simulink model "KF"  (R2021a)
settings: Solver=ode45  StartTime=0.0  StopTime=tt(end)  MaxStep=0.1  RelTol=1e-3  EnableMultiTasking=on
model workspace (MATLAB code in the model file + MAT data in the model file):
  L = 2.5
  v0 = 0
  xe0 = 0
  xn0 = 0
  theta0 = 0
  Ts = 1
  rr = [0 0 0 0 0 0 0 0 0 0 0 0 ... (9404 elements, 9404x1)]
  tt = [0 0.05 0.1 0.15 0.2 0.25 0.3 0.35 0.4 0.45 0.5 0.55 ... (9404 elements, 9404x1)]
  vv = [25 25 25 25 25 25 25 25 25 25 25 25 ... (9404 elements, 9404x1)]
undefined symbols (not defined in the file or in its folder): Discrete, Time
libraries: simulink x4, pid_lib x2, ctrlSharedLib x1
(part 2 of 2)

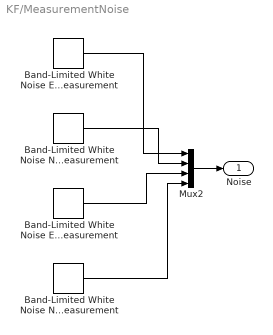
== system KF/MeasurementNoise ==
  Band-Limited White Noise North Position Measurement : simulink/Sources/Band-Limited White Noise  Cov=50  Ts=Ts  seed=[23342]
  Band-Limited White Noise North Velocity Measurement : simulink/Sources/Band-Limited White Noise  Cov=50  Ts=Ts  seed=[23342]
  Band-Limited White Noise East Position Measurement : simulink/Sources/Band-Limited White Noise  Cov=50  Ts=Ts  seed=[23341]
  Band-Limited White Noise East Velocity Measurement : simulink/Sources/Band-Limited White Noise  Cov=50  Ts=Ts  seed=[23341]
  Mux2 : Mux
  Noise : Outport
  wires:
  Mux2/1 -> Noise/1
  Band-Limited White Noise East Position Measurement/1 -> Mux2/1
  Band-Limited White Noise North Position Measurement/1 -> Mux2/2
  Band-Limited White Noise East Velocity Measurement/1 -> Mux2/3
  Band-Limited White Noise North Velocity Measurement/1 -> Mux2/4

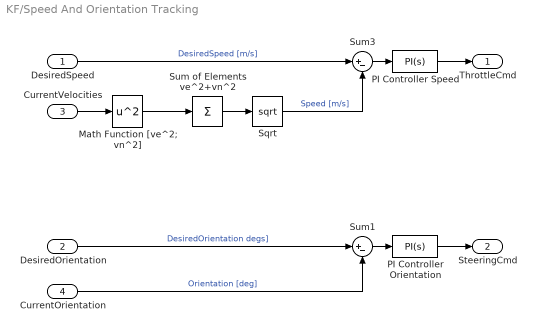
== system KF/Speed And Orientation Tracking ==
  DesiredSpeed : Inport
  DesiredOrientation : Inport  Port=2
  CurrentVelocities : Inport  Port=3
  CurrentOrientation : Inport  Port=4
  Math Function [ve^2; vn^2] : Math  Operator=square  SignedPower=on  SaturateOnIntegerOverflow=on
  PI Controller Orientation : pid_lib/PID Controller  Controller=PI  Form=Parallel  TimeDomain=Continuous-time  UseExternalTs=off  SampleTime=-1  IntegratorMethod=Forward Euler  FilterMethod=Forward Euler  ControllerParametersSource=internal  P=1  I=0.3  D=0  UseFilter=on  N=100  TunerSelectOption=Transfer Function Based (PID Tuner App)  InitialConditionSource=internal  InitialConditionForIntegrator=0  InitialConditionForFilter=0  DifferentiatorICPrevScaledInput=0  ExternalReset=none  TrackingMode=off  Kt=1  LimitOutput=on  SatLimitsSource=internal  UpperSaturationLimit=20  LowerSaturationLimit=-20  LinearizeAsGain=off  AntiWindupMode=clamping  Kb=1  POutMin=[]  POutMax=[]  IOutMin=[]  IOutMax=[]  DOutMin=[]  DOutMax=[]  NOutMin=[]  NOutMax=[]  SumOutMin=[]  SumOutMax=[]  SaturationOutMin=[]  SaturationOutMax=[]  PParamMin=[]  PParamMax=[]  IParamMin=[]  IParamMax=[]  DParamMin=[]  DParamMax=[]  NParamMin=[]  NParamMax=[]  KbParamMin=[]  KbParamMax=[]  KtParamMin=[]  KtParamMax=[]  KbOutMin=[]  KbOutMax=[]  KtOutMin=[]  KtOutMax=[]  IntegratorOutMin=[]  IntegratorOutMax=[]  FilterOutMin=[]  FilterOutMax=[]  SumI1OutMin=[]  SumI1OutMax=[]  SumI2OutMin=[]  SumI2OutMax=[]  SumI3OutMin=[]  SumI3OutMax=[]  SumI4OutMin=[]  SumI4OutMax=[]  SumDOutMin=[]  SumDOutMax=[]  DifferentiatorOutMin=[]  DifferentiatorOutMax=[]  FilterDiffOutCoefMin=[]  FilterDiffOutCoefMax=[]  ReciprocalOutMin=[]  ReciprocalOutMax=[]  SumDenOutMin=[]  SumDenOutMax=[]  SumNumOutMin=[]  SumNumOutMax=[]  DivideOutMin=[]  DivideOutMax=[]  UdiffTsProdOutMin=[]  UdiffTsProdOutMax=[]  NTsProdOutMin=[]  NTsProdOutMax=[]  UintegralTsProdOutMin=[]  UintegralTsProdOutMax=[]  UngainTsProdOutMin=[]  UngainTsProdOutMax=[]  IntegratorContinuousStateAttributes=''  IntegratorStateMustResolveToSignalObject=off  IntegratorRTWStateStorageClass=Auto  FilterContinuousStateAttributes=''  FilterStateMustResolveToSignalObject=off  FilterRTWStateStorageClass=Auto  ParallelPVariant=InternalParameters  IdealPVariant=Disabled  IVariant=InternalParameters  DVariant=Disabled  IntegratorVariant=Continuous  SatVariant=Enabled  AWVariant=ContClampingParallel  PCopyVariant=Disabled  TRVariant=Disabled  FdbkBlocksVariant=Forward  IdealPFdbkVariant=Disabled  SatFdbkVariant=Disabled  DerivativeFilterVariant=Disabled  NVariant=Disabled  NCopyVariant=Disabled_SignalSpec  FilterICVariant=Disabled  IntegratorICVariant=InternalICs  ExternalResetVariant=Disabled  TRSumVariant=Passthrough  SumFdbkVariant=Disabled  SumVariant=Sum_PI  TsampFilterVariant=InternalTs  TsampNgainVariant=Passthrough  TsampIntegralVariant=Passthrough  ExternalSaturationOutDataTypeStr=Inherit: Same as second input
  PI Controller Speed : pid_lib/PID Controller  Controller=PI  Form=Parallel  TimeDomain=Continuous-time  UseExternalTs=off  SampleTime=-1  IntegratorMethod=Forward Euler  FilterMethod=Forward Euler  ControllerParametersSource=internal  P=0.15  I=0.01  D=0  UseFilter=on  N=100  TunerSelectOption=Transfer Function Based (PID Tuner App)  InitialConditionSource=internal  InitialConditionForIntegrator=0  InitialConditionForFilter=0  DifferentiatorICPrevScaledInput=0  ExternalReset=none  TrackingMode=off  Kt=1  LimitOutput=on  SatLimitsSource=internal  UpperSaturationLimit=1  LowerSaturationLimit=-1  LinearizeAsGain=off  AntiWindupMode=clamping  Kb=1  POutMin=[]  POutMax=[]  IOutMin=[]  IOutMax=[]  DOutMin=[]  DOutMax=[]  NOutMin=[]  NOutMax=[]  SumOutMin=[]  SumOutMax=[]  SaturationOutMin=[]  SaturationOutMax=[]  PParamMin=[]  PParamMax=[]  IParamMin=[]  IParamMax=[]  DParamMin=[]  DParamMax=[]  NParamMin=[]  NParamMax=[]  KbParamMin=[]  KbParamMax=[]  KtParamMin=[]  KtParamMax=[]  KbOutMin=[]  KbOutMax=[]  KtOutMin=[]  KtOutMax=[]  IntegratorOutMin=[]  IntegratorOutMax=[]  FilterOutMin=[]  FilterOutMax=[]  SumI1OutMin=[]  SumI1OutMax=[]  SumI2OutMin=[]  SumI2OutMax=[]  SumI3OutMin=[]  SumI3OutMax=[]  SumI4OutMin=[]  SumI4OutMax=[]  SumDOutMin=[]  SumDOutMax=[]  DifferentiatorOutMin=[]  DifferentiatorOutMax=[]  FilterDiffOutCoefMin=[]  FilterDiffOutCoefMax=[]  ReciprocalOutMin=[]  ReciprocalOutMax=[]  SumDenOutMin=[]  SumDenOutMax=[]  SumNumOutMin=[]  SumNumOutMax=[]  DivideOutMin=[]  DivideOutMax=[]  UdiffTsProdOutMin=[]  UdiffTsProdOutMax=[]  NTsProdOutMin=[]  NTsProdOutMax=[]  UintegralTsProdOutMin=[]  UintegralTsProdOutMax=[]  UngainTsProdOutMin=[]  UngainTsProdOutMax=[]  IntegratorContinuousStateAttributes=''  IntegratorStateMustResolveToSignalObject=off  IntegratorRTWStateStorageClass=Auto  FilterContinuousStateAttributes=''  FilterStateMustResolveToSignalObject=off  FilterRTWStateStorageClass=Auto  ParallelPVariant=InternalParameters  IdealPVariant=Disabled  IVariant=InternalParameters  DVariant=Disabled  IntegratorVariant=Continuous  SatVariant=Enabled  AWVariant=ContClampingParallel  PCopyVariant=Disabled  TRVariant=Disabled  FdbkBlocksVariant=Forward  IdealPFdbkVariant=Disabled  SatFdbkVariant=Disabled  DerivativeFilterVariant=Disabled  NVariant=Disabled  NCopyVariant=Disabled_SignalSpec  FilterICVariant=Disabled  IntegratorICVariant=InternalICs  ExternalResetVariant=Disabled  TRSumVariant=Passthrough  SumFdbkVariant=Disabled  SumVariant=Sum_PI  TsampFilterVariant=InternalTs  TsampNgainVariant=Passthrough  TsampIntegralVariant=Passthrough  ExternalSaturationOutDataTypeStr=Inherit: Same as second input
  Sqrt : Sqrt  SaturateOnIntegerOverflow=on
  Sum of Elements ve^2+vn^2 : Sum  Inputs=+
  Sum1 : Sum  Inputs=|+-
  Sum3 : Sum  Inputs=|+-
  ThrottleCmd : Outport
  SteeringCmd : Outport  Port=2
  wires:
  PI Controller Speed/1 -> ThrottleCmd/1
  DesiredSpeed/1 -> Sum3/1  "DesiredSpeed [m/s]"
  Sum3/1 -> PI Controller Speed/1
  CurrentVelocities/1 -> Math Function [ve^2; vn^2]/1
  Math Function [ve^2; vn^2]/1 -> Sum of Elements ve^2+vn^2/1
  Sum of Elements ve^2+vn^2/1 -> Sqrt/1
  Sqrt/1 -> Sum3/2  "Speed [m/s]"
  PI Controller Orientation/1 -> SteeringCmd/1
  DesiredOrientation/1 -> Sum1/1  "DesiredOrientation degs]"
  Sum1/1 -> PI Controller Orientation/1
  CurrentOrientation/1 -> Sum1/2  "Orientation [deg]"

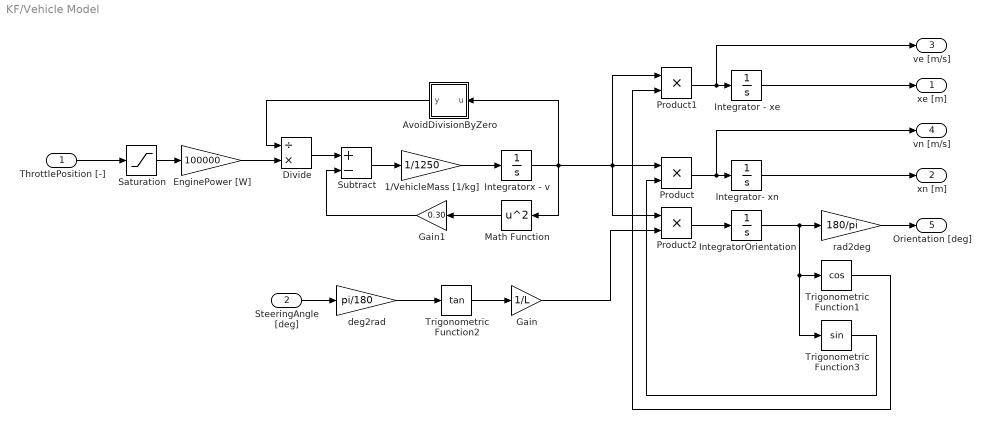
== system KF/Vehicle Model ==
  ThrottlePosition [-] : Inport
  "SteeringAngle [deg] " : Inport  Port=2
  1/VehicleMass [1/kg] : Gain  Gain=1/1250
  AvoidDivisionByZero : Subsystem
  Divide : Product  Inputs=/*
  EnginePower [W] : Gain  Gain=100000
  Gain : Gain  Gain=1/L
  Gain1 : Gain  Gain=0.30
  Integrator - xe : Integrator  InitialCondition=xe0
  Integrator- xn : Integrator  InitialCondition=xn0
  IntegratorOrientation : Integrator  InitialCondition=theta0
  Integratorx - v : Integrator  InitialCondition=v0
  Math Function : Math  Operator=square  SignedPower=on  SaturateOnIntegerOverflow=on
  Product : Product
  Product1 : Product
  Product2 : Product
  Saturation : Saturate  UpperLimit=1  LowerLimit=-1
  Subtract : Sum  Inputs=+-
  Trigonometric Function1 : Trigonometry  Operator=cos
  Trigonometric Function2 : Trigonometry  Operator=tan
  Trigonometric Function3 : Trigonometry
  deg2rad : Gain  Gain=pi/180
  rad2deg : Gain  Gain=180/pi
  xe [m] : Outport
  xn [m] : Outport  Port=2
  ve [m/s] : Outport  Port=3
  vn [m/s] : Outport  Port=4
  Orientation [deg] : Outport  Port=5
  wires:
  Trigonometric Function3/1 -> Product/2
  Product/1 -> vn [m/s]/1, Integrator- xn/1
  Product1/1 -> ve [m/s]/1, Integrator - xe/1
  Product2/1 -> IntegratorOrientation/1
  "SteeringAngle [deg] "/1 -> deg2rad/1
  Gain/1 -> Product2/2
  Trigonometric Function2/1 -> Gain/1
  Integrator - xe/1 -> xe [m]/1
  Integrator- xn/1 -> xn [m]/1
  IntegratorOrientation/1 -> Trigonometric Function3/1, Trigonometric Function1/1, rad2deg/1
  deg2rad/1 -> Trigonometric Function2/1
  rad2deg/1 -> Orientation [deg]/1
  ThrottlePosition [-]/1 -> Saturation/1
  Integratorx - v/1 -> Math Function/1, AvoidDivisionByZero/1(u), Product1/1, Product/1, Product2/1
  Saturation/1 -> EnginePower [W]/1
  EnginePower [W]/1 -> Divide/2
  AvoidDivisionByZero/1(y) -> Divide/1
  Trigonometric Function1/1 -> Product1/2
  Divide/1 -> Subtract/1
  Subtract/1 -> 1/VehicleMass [1/kg]/1
  Math Function/1 -> Gain1/1
  Gain1/1 -> Subtract/2
  1/VehicleMass [1/kg]/1 -> Integratorx - v/1

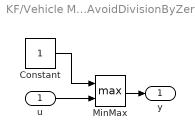
== system KF/Vehicle Model/AvoidDivisionByZero ==
  u : Inport
  Constant : Constant
  MinMax : MinMax  Function=max  Inputs=2
  y : Outport
  wires:
  MinMax/1 -> y/1
  Constant/1 -> MinMax/1
  u/1 -> MinMax/2
